simulink model "linear_motor_zs"  (R2017b)
settings: Solver=FixedStepAuto  StartTime=0.0  StopTime=200  FixedStep=1e-3  RelTol=1e-3
values from neighbouring files (symbols this model uses):
  J_ind = 4.1    [linear_motor_params.m]    (also in robust_linear_motor_params.m = ureal('J_ind',4.1,'Percentage',range); ship_induction_motor_propulsion_extended_linear.m)
  L_ad_ind = L_aq_ind    (= 0.00307086614173)    [linear_motor_params.m]    (also in robust_linear_motor_params.m = L_aq_ind; ship_induction_motor_propulsion_extended_linear.m)
  L_aq_ind = 1/(1/L_M_ind + 1/L_ls_ind + 1/L_lr_ind)    (= 0.00307086614173)    [linear_motor_params.m]    (also in robust_linear_motor_params.m = 1/(1/L_M_ind + 1/L_ls_ind + 1/L_lr_ind); ship_induction_motor_propulsion_extended_linear.m)
  L_eq = L_ls_ind + L_M_ind *(L_lr_ind)/(L_lr_ind+L_M_ind)    (= 0.0188613861386)    [linear_motor_params.m]    (also in robust_linear_motor_params.m = L_ls_ind + L_M_ind *(L_lr_ind)/(L_lr_ind+L_M_ind); ship_induction_motor_propulsion_extended_linear.m)
  L_lr_ind = 15e-3    (= 0.015)    [linear_motor_params.m]    (also in robust_linear_motor_params.m = ureal('L_lr_ind',15e-3, 'Percentage',range); ship_induction_motor_propulsion_extended_linear.m)
  L_ls_ind = 15e-3    (= 0.015)    [linear_motor_params.m]    (also in robust_linear_motor_params.m = ureal('L_ls_ind',15e-3, 'Percentage',range); ship_induction_motor_propulsion_extended_linear.m)
  L_M_ind = 5.2e-3    (= 0.0052)    [linear_motor_params.m]    (also in robust_linear_motor_params.m = ureal('L_M_ind',5.2e-3, 'Percentage',range); ship_induction_motor_propulsion_extended_linear.m)
  P_ind = 4    [linear_motor_params.m]    (also in robust_linear_motor_params.m; ship_induction_motor_propulsion_extended_linear.m)
  r_r_ind = 4.6e-3    (= 0.0046)    [linear_motor_params.m]    (also in robust_linear_motor_params.m = ureal('r_r_ind', 4.6e-3, 'Percentage', range); ship_induction_motor_propulsion_extended_linear.m)
  r_s_ind = 7.6e-3    (= 0.0076)    [linear_motor_params.m]    (also in robust_linear_motor_params.m = ureal('r_s_ind', 7.6e-3, 'Percentage', range); ship_induction_motor_propulsion_extended_linear.m)
  T_r_ind = L_lr_ind/r_r_ind    (= 3.26086956522)    [linear_motor_params.m]    (also in robust_linear_motor_params.m = L_lr_ind/r_r_ind; ship_induction_motor_propulsion_extended_linear.m)
  T_s_est = 1e-2    (= 0.01)    [linear_motor_params.m]    (also in robust_linear_motor_params.m; ship_induction_motor_propulsion_extended_linear.m)
  Ts = 1e-3    (= 0.001)    [linear_motor_params.m]    (also in robust_linear_motor_params.m; ship_induction_motor_propulsion_extended_linear.m)
libraries: simulink x6, cstblocks x2
settings Model: Creator=z003vh9b  LastModifiedBy=zhensong
settings CodeAppCC: StateflowObjectComments=on

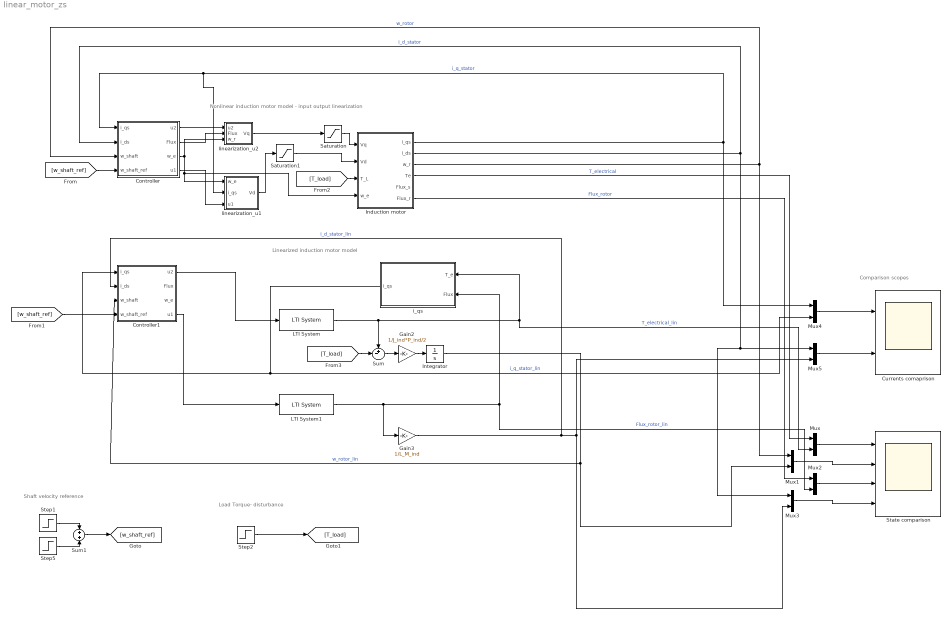
== system linear_motor_zs ==
  note: Comparison scopes
  note: Linearized induction motor model
  note: Nonlinear induction motor model - input output linearization
  note: Load Torque- disturbance
  note: Shaft velocity reference
  Controller : Subsystem
  Controller1 : Subsystem
  Currents comaprison : Scope  NumInputPorts=2
  Gain2 : Gain  Gain=1/J_ind*P_ind/2
  Gain3 : Gain  Gain=1/L_M_ind
  Induction motor : Subsystem
  Integrator : Integrator
  LTI System : cstblocks/LTI System  sys=G_torque  IC=[]  mask(LTI Block){}
  LTI System1 : cstblocks/LTI System  sys=G_flux  IC=[]
  Mux{,1..5} (6 alike) : Mux  Inputs=2
  Saturation : Saturate  UpperLimit=500  LowerLimit=-500
  Saturation1 : Saturate  UpperLimit=500  LowerLimit=-500
  State comparison : Scope  NumInputPorts=4
  Step1 : Step  Time=50  SampleTime=0
  Step2 : Step  Time=100  After=10  SampleTime=0
  Step5 : Step  Time=180  After=-2  SampleTime=0
  Sum : Sum  Inputs=+-|
  Sum1 : Sum
  i_qs : Subsystem
  linearization_u1 : Subsystem
  linearization_u2 : Subsystem
  wires:
  Induction motor/3(w_r) -> Mux1/1, Controller/3(w_shaft)  "w_rotor"
  Induction motor/4(Te) -> Mux/1  "T_electrical"
  Induction motor/2(i_ds) -> Mux3/1, Mux5/1, Controller/2(i_ds)  "i_d_stator"
  Induction motor/1(i_qs) -> Mux4/1, linearization_u1/2(i_qs), Controller/1(i_qs)  "i_q_stator"
  linearization_u2/1(Vq) -> Saturation/1
  linearization_u1/1(Vd) -> Saturation1/1
  Mux/1 -> State comparison/1
  Mux1/1 -> State comparison/2
  Mux2/1 -> State comparison/3
  Mux3/1 -> State comparison/4
  LTI System1/1 -> i_qs/2(Flux), Mux2/2, Gain3/1  "Flux_rotor_lin"
  Gain3/1 -> Mux3/2, Mux5/2, Controller1/2(i_ds)  "i_d_stator_lin"
  Induction motor/6(Flux_r) -> Mux2/1  "Flux_rotor"
  Step5/1 -> Sum1/2
  Step1/1 -> Sum1/1
  [w_shaft_ref] -> Controller/4(w_shaft_ref)
  Saturation/1 -> Induction motor/1(Vq)
  Saturation1/1 -> Induction motor/2(Vd)
  LTI System/1 -> Sum/1, i_qs/1(T_e), Mux/2  "T_electrical_lin"
  Integrator/1 -> Mux1/2, Controller1/3(w_shaft)  "w_rotor_lin"
  Gain2/1 -> Integrator/1
  Controller/1(u2) -> linearization_u2/1(u2)
  Controller/2(Flux) -> linearization_u2/2(Flux)
  Controller/3(w_e) -> linearization_u2/3(w_r), linearization_u1/1(w_e), Induction motor/4(w_e)
  Controller/4(u1) -> linearization_u1/3(u1)
  Controller1/4(u1) -> LTI System1/1
  Controller1/1(u2) -> LTI System/1
  i_qs/1(i_qs) -> Controller1/1(i_qs), Mux4/2  "i_q_stator_lin"
  Sum1/1 -> [w_shaft_ref]
  [w_shaft_ref] -> Controller1/4(w_shaft_ref)
  Step2/1 -> [T_load]
  [T_load] -> Induction motor/3(T_L)
  [T_load] -> Sum/2
  Sum/1 -> Gain2/1
  Mux4/1 -> Currents comaprison/1
  Mux5/1 -> Currents comaprison/2

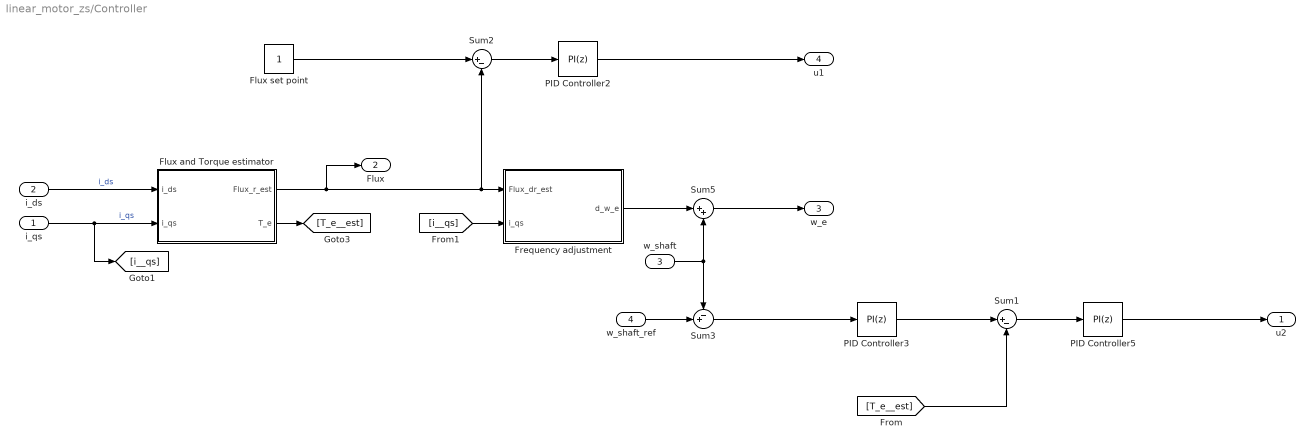
== system linear_motor_zs/Controller ==
  i_qs : Inport
  i_ds : Inport  Port=2
  w_shaft : Inport  Port=3
  w_shaft_ref : Inport  Port=4
  Flux and Torque estimator : Subsystem
  Flux set point : Constant
  Frequency adjustment : Subsystem
  PID Controller2 : simulink/Continuous/PID Controller  Controller=PI  TimeDomain=Discrete-time  SampleTime=0.01  IntegratorMethod=Forward Euler  FilterMethod=Forward Euler  Form=Parallel  UseFilter=on  ControllerParametersSource=internal  P=1  I=0.1  D=0  N=100  InitialConditionSource=internal  InitialConditionForIntegrator=0  InitialConditionForFilter=0  ExternalReset=none  LimitOutput=off  UpperSaturationLimit=inf  LowerSaturationLimit=-inf  LinearizeAsGain=on  AntiWindupMode=none  Kb=1  TrackingMode=off  Kt=1  PParamMin=[]  PParamMax=[]  IParamMin=[]  IParamMax=[]  DParamMin=[]  DParamMax=[]  NParamMin=[]  NParamMax=[]  KbParamMin=[]  KbParamMax=[]  KtParamMin=[]  KtParamMax=[]  POutMin=[]  POutMax=[]  IOutMin=[]  IOutMax=[]  DOutMin=[]  DOutMax=[]  NOutMin=[]  NOutMax=[]  KbOutMin=[]  KbOutMax=[]  KtOutMin=[]  KtOutMax=[]  IntegratorOutMin=[]  IntegratorOutMax=[]  FilterOutMin=[]  FilterOutMax=[]  SumOutMin=[]  SumOutMax=[]  SumI1OutMin=[]  SumI1OutMax=[]  SumI2OutMin=[]  SumI2OutMax=[]  SumI3OutMin=[]  SumI3OutMax=[]  SumDOutMin=[]  SumDOutMax=[]  SaturationOutMin=[]  SaturationOutMax=[]  IntegratorContinuousStateAttributes=''  IntegratorStateMustResolveToSignalObject=off  IntegratorRTWStateStorageClass=Auto  FilterContinuousStateAttributes=''  FilterStateMustResolveToSignalObject=off  FilterRTWStateStorageClass=Auto  DifferentiatorICPrevScaledInput=0  DifferentiatorOutMin=[]  DifferentiatorOutMax=[]  InitialConditionSetting=State (most efficient)  FilterDiffOutCoefMin=[]  FilterDiffOutCoefMax=[]  SumDenOutMin=[]  SumDenOutMax=[]  SumNumOutMin=[]  SumNumOutMax=[]  ReciprocalOutMin=[]  ReciprocalOutMax=[]  DivideOutMin=[]  DivideOutMax=[]  TunerSelectOption=Transfer Function Based (PID Tuner App)
  PID Controller3 : simulink/Continuous/PID Controller  Controller=PI  TimeDomain=Discrete-time  SampleTime=Ts  IntegratorMethod=Forward Euler  FilterMethod=Forward Euler  Form=Parallel  UseFilter=on  ControllerParametersSource=internal  P=10  I=10  D=1  N=100  InitialConditionSource=internal  InitialConditionForIntegrator=0  InitialConditionForFilter=0  ExternalReset=none  LimitOutput=off  UpperSaturationLimit=inf  LowerSaturationLimit=-inf  LinearizeAsGain=on  AntiWindupMode=none  Kb=1  TrackingMode=off  Kt=1  PParamMin=[]  PParamMax=[]  IParamMin=[]  IParamMax=[]  DParamMin=[]  DParamMax=[]  NParamMin=[]  NParamMax=[]  KbParamMin=[]  KbParamMax=[]  KtParamMin=[]  KtParamMax=[]  POutMin=[]  POutMax=[]  IOutMin=[]  IOutMax=[]  DOutMin=[]  DOutMax=[]  NOutMin=[]  NOutMax=[]  KbOutMin=[]  KbOutMax=[]  KtOutMin=[]  KtOutMax=[]  IntegratorOutMin=[]  IntegratorOutMax=[]  FilterOutMin=[]  FilterOutMax=[]  SumOutMin=[]  SumOutMax=[]  SumI1OutMin=[]  SumI1OutMax=[]  SumI2OutMin=[]  SumI2OutMax=[]  SumI3OutMin=[]  SumI3OutMax=[]  SumDOutMin=[]  SumDOutMax=[]  SaturationOutMin=[]  SaturationOutMax=[]  IntegratorContinuousStateAttributes=''  IntegratorStateMustResolveToSignalObject=off  IntegratorRTWStateStorageClass=Auto  FilterContinuousStateAttributes=''  FilterStateMustResolveToSignalObject=off  FilterRTWStateStorageClass=Auto  DifferentiatorICPrevScaledInput=0  DifferentiatorOutMin=[]  DifferentiatorOutMax=[]  InitialConditionSetting=State (most efficient)  FilterDiffOutCoefMin=[]  FilterDiffOutCoefMax=[]  SumDenOutMin=[]  SumDenOutMax=[]  SumNumOutMin=[]  SumNumOutMax=[]  ReciprocalOutMin=[]  ReciprocalOutMax=[]  DivideOutMin=[]  DivideOutMax=[]  TunerSelectOption=Transfer Function Based (PID Tuner App)
  PID Controller5 : simulink/Continuous/PID Controller  Controller=PI  TimeDomain=Discrete-time  SampleTime=Ts  IntegratorMethod=Forward Euler  FilterMethod=Forward Euler  Form=Parallel  UseFilter=on  ControllerParametersSource=internal  P=1  I=10  D=1  N=100  InitialConditionSource=internal  InitialConditionForIntegrator=0  InitialConditionForFilter=0  ExternalReset=none  LimitOutput=off  UpperSaturationLimit=500  LowerSaturationLimit=-500  LinearizeAsGain=on  AntiWindupMode=none  Kb=1  TrackingMode=off  Kt=1  PParamMin=[]  PParamMax=[]  IParamMin=[]  IParamMax=[]  DParamMin=[]  DParamMax=[]  NParamMin=[]  NParamMax=[]  KbParamMin=[]  KbParamMax=[]  KtParamMin=[]  KtParamMax=[]  POutMin=[]  POutMax=[]  IOutMin=[]  IOutMax=[]  DOutMin=[]  DOutMax=[]  NOutMin=[]  NOutMax=[]  KbOutMin=[]  KbOutMax=[]  KtOutMin=[]  KtOutMax=[]  IntegratorOutMin=[]  IntegratorOutMax=[]  FilterOutMin=[]  FilterOutMax=[]  SumOutMin=[]  SumOutMax=[]  SumI1OutMin=[]  SumI1OutMax=[]  SumI2OutMin=[]  SumI2OutMax=[]  SumI3OutMin=[]  SumI3OutMax=[]  SumDOutMin=[]  SumDOutMax=[]  SaturationOutMin=[]  SaturationOutMax=[]  IntegratorContinuousStateAttributes=''  IntegratorStateMustResolveToSignalObject=off  IntegratorRTWStateStorageClass=Auto  FilterContinuousStateAttributes=''  FilterStateMustResolveToSignalObject=off  FilterRTWStateStorageClass=Auto  DifferentiatorICPrevScaledInput=0  DifferentiatorOutMin=[]  DifferentiatorOutMax=[]  InitialConditionSetting=State (most efficient)  FilterDiffOutCoefMin=[]  FilterDiffOutCoefMax=[]  SumDenOutMin=[]  SumDenOutMax=[]  SumNumOutMin=[]  SumNumOutMax=[]  ReciprocalOutMin=[]  ReciprocalOutMax=[]  DivideOutMin=[]  DivideOutMax=[]  TunerSelectOption=Transfer Function Based (PID Tuner App)
  Sum1 : Sum  Inputs=|+-
  Sum2 : Sum  Inputs=|+-
  Sum3 : Sum  Inputs=-+|
  Sum5 : Sum  Inputs=|++
  u2 : Outport
  Flux : Outport  Port=2
  w_e : Outport  Port=3
  u1 : Outport  Port=4
  wires:
  Sum2/1 -> PID Controller2/1
  Sum5/1 -> w_e/1
  Flux and Torque estimator/1(Flux_r_est) -> Flux/1, Frequency adjustment/1(Flux_dr_est), Sum2/2
  w_shaft/1 -> Sum3/1, Sum5/2
  Frequency adjustment/1(d_w_e) -> Sum5/1
  Flux set point/1 -> Sum2/1
  Sum3/1 -> PID Controller3/1
  [i__qs] -> Frequency adjustment/2(i_qs)
  i_ds/1 -> Flux and Torque estimator/1(i_ds)  "i_ds"
  i_qs/1 -> Flux and Torque estimator/2(i_qs), [i__qs]  "i_qs"
  Sum1/1 -> PID Controller5/1
  Flux and Torque estimator/2(T_e) -> [T_e__est]
  PID Controller3/1 -> Sum1/1
  [T_e__est] -> Sum1/2
  PID Controller2/1 -> u1/1
  PID Controller5/1 -> u2/1
  w_shaft_ref/1 -> Sum3/2

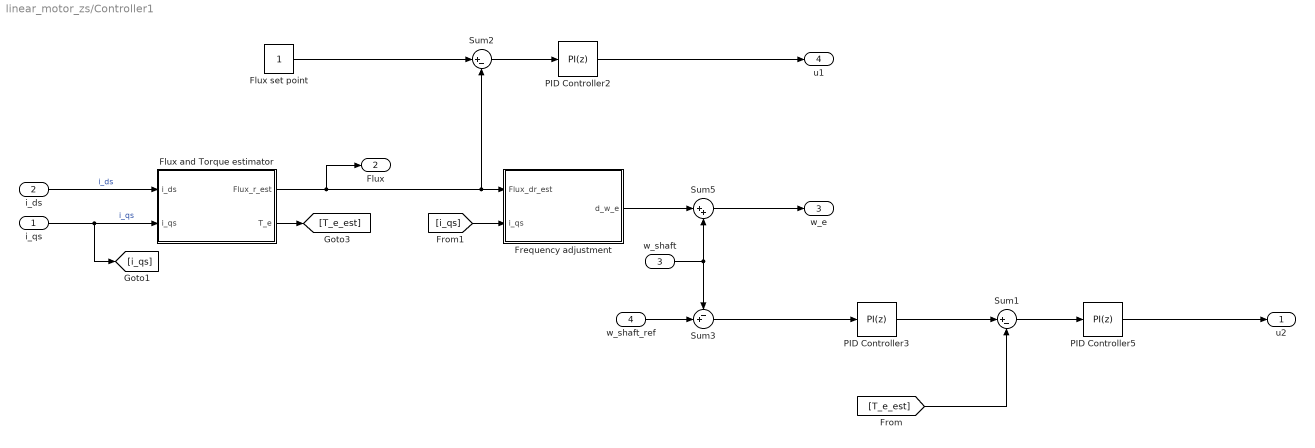
== system linear_motor_zs/Controller1 ==
  i_qs : Inport
  i_ds : Inport  Port=2
  w_shaft : Inport  Port=3
  w_shaft_ref : Inport  Port=4
  Flux and Torque estimator : Subsystem
  Flux set point : Constant
  Frequency adjustment : Subsystem
  PID Controller2 : simulink/Continuous/PID Controller  Controller=PI  TimeDomain=Discrete-time  SampleTime=0.01  IntegratorMethod=Forward Euler  FilterMethod=Forward Euler  Form=Parallel  UseFilter=on  ControllerParametersSource=internal  P=1  I=0.1  D=0  N=100  InitialConditionSource=internal  InitialConditionForIntegrator=0  InitialConditionForFilter=0  ExternalReset=none  LimitOutput=off  UpperSaturationLimit=inf  LowerSaturationLimit=-inf  LinearizeAsGain=on  AntiWindupMode=none  Kb=1  TrackingMode=off  Kt=1  PParamMin=[]  PParamMax=[]  IParamMin=[]  IParamMax=[]  DParamMin=[]  DParamMax=[]  NParamMin=[]  NParamMax=[]  KbParamMin=[]  KbParamMax=[]  KtParamMin=[]  KtParamMax=[]  POutMin=[]  POutMax=[]  IOutMin=[]  IOutMax=[]  DOutMin=[]  DOutMax=[]  NOutMin=[]  NOutMax=[]  KbOutMin=[]  KbOutMax=[]  KtOutMin=[]  KtOutMax=[]  IntegratorOutMin=[]  IntegratorOutMax=[]  FilterOutMin=[]  FilterOutMax=[]  SumOutMin=[]  SumOutMax=[]  SumI1OutMin=[]  SumI1OutMax=[]  SumI2OutMin=[]  SumI2OutMax=[]  SumI3OutMin=[]  SumI3OutMax=[]  SumDOutMin=[]  SumDOutMax=[]  SaturationOutMin=[]  SaturationOutMax=[]  IntegratorContinuousStateAttributes=''  IntegratorStateMustResolveToSignalObject=off  IntegratorRTWStateStorageClass=Auto  FilterContinuousStateAttributes=''  FilterStateMustResolveToSignalObject=off  FilterRTWStateStorageClass=Auto  DifferentiatorICPrevScaledInput=0  DifferentiatorOutMin=[]  DifferentiatorOutMax=[]  InitialConditionSetting=State (most efficient)  FilterDiffOutCoefMin=[]  FilterDiffOutCoefMax=[]  SumDenOutMin=[]  SumDenOutMax=[]  SumNumOutMin=[]  SumNumOutMax=[]  ReciprocalOutMin=[]  ReciprocalOutMax=[]  DivideOutMin=[]  DivideOutMax=[]  TunerSelectOption=Transfer Function Based (PID Tuner App)
  PID Controller3 : simulink/Continuous/PID Controller  Controller=PI  TimeDomain=Discrete-time  SampleTime=Ts  IntegratorMethod=Forward Euler  FilterMethod=Forward Euler  Form=Parallel  UseFilter=on  ControllerParametersSource=internal  P=10  I=10  D=1  N=100  InitialConditionSource=internal  InitialConditionForIntegrator=0  InitialConditionForFilter=0  ExternalReset=none  LimitOutput=off  UpperSaturationLimit=inf  LowerSaturationLimit=-inf  LinearizeAsGain=on  AntiWindupMode=none  Kb=1  TrackingMode=off  Kt=1  PParamMin=[]  PParamMax=[]  IParamMin=[]  IParamMax=[]  DParamMin=[]  DParamMax=[]  NParamMin=[]  NParamMax=[]  KbParamMin=[]  KbParamMax=[]  KtParamMin=[]  KtParamMax=[]  POutMin=[]  POutMax=[]  IOutMin=[]  IOutMax=[]  DOutMin=[]  DOutMax=[]  NOutMin=[]  NOutMax=[]  KbOutMin=[]  KbOutMax=[]  KtOutMin=[]  KtOutMax=[]  IntegratorOutMin=[]  IntegratorOutMax=[]  FilterOutMin=[]  FilterOutMax=[]  SumOutMin=[]  SumOutMax=[]  SumI1OutMin=[]  SumI1OutMax=[]  SumI2OutMin=[]  SumI2OutMax=[]  SumI3OutMin=[]  SumI3OutMax=[]  SumDOutMin=[]  SumDOutMax=[]  SaturationOutMin=[]  SaturationOutMax=[]  IntegratorContinuousStateAttributes=''  IntegratorStateMustResolveToSignalObject=off  IntegratorRTWStateStorageClass=Auto  FilterContinuousStateAttributes=''  FilterStateMustResolveToSignalObject=off  FilterRTWStateStorageClass=Auto  DifferentiatorICPrevScaledInput=0  DifferentiatorOutMin=[]  DifferentiatorOutMax=[]  InitialConditionSetting=State (most efficient)  FilterDiffOutCoefMin=[]  FilterDiffOutCoefMax=[]  SumDenOutMin=[]  SumDenOutMax=[]  SumNumOutMin=[]  SumNumOutMax=[]  ReciprocalOutMin=[]  ReciprocalOutMax=[]  DivideOutMin=[]  DivideOutMax=[]  TunerSelectOption=Transfer Function Based (PID Tuner App)
  PID Controller5 : simulink/Continuous/PID Controller  Controller=PI  TimeDomain=Discrete-time  SampleTime=Ts  IntegratorMethod=Forward Euler  FilterMethod=Forward Euler  Form=Parallel  UseFilter=on  ControllerParametersSource=internal  P=1  I=10  D=1  N=100  InitialConditionSource=internal  InitialConditionForIntegrator=0  InitialConditionForFilter=0  ExternalReset=none  LimitOutput=off  UpperSaturationLimit=500  LowerSaturationLimit=-500  LinearizeAsGain=on  AntiWindupMode=none  Kb=1  TrackingMode=off  Kt=1  PParamMin=[]  PParamMax=[]  IParamMin=[]  IParamMax=[]  DParamMin=[]  DParamMax=[]  NParamMin=[]  NParamMax=[]  KbParamMin=[]  KbParamMax=[]  KtParamMin=[]  KtParamMax=[]  POutMin=[]  POutMax=[]  IOutMin=[]  IOutMax=[]  DOutMin=[]  DOutMax=[]  NOutMin=[]  NOutMax=[]  KbOutMin=[]  KbOutMax=[]  KtOutMin=[]  KtOutMax=[]  IntegratorOutMin=[]  IntegratorOutMax=[]  FilterOutMin=[]  FilterOutMax=[]  SumOutMin=[]  SumOutMax=[]  SumI1OutMin=[]  SumI1OutMax=[]  SumI2OutMin=[]  SumI2OutMax=[]  SumI3OutMin=[]  SumI3OutMax=[]  SumDOutMin=[]  SumDOutMax=[]  SaturationOutMin=[]  SaturationOutMax=[]  IntegratorContinuousStateAttributes=''  IntegratorStateMustResolveToSignalObject=off  IntegratorRTWStateStorageClass=Auto  FilterContinuousStateAttributes=''  FilterStateMustResolveToSignalObject=off  FilterRTWStateStorageClass=Auto  DifferentiatorICPrevScaledInput=0  DifferentiatorOutMin=[]  DifferentiatorOutMax=[]  InitialConditionSetting=State (most efficient)  FilterDiffOutCoefMin=[]  FilterDiffOutCoefMax=[]  SumDenOutMin=[]  SumDenOutMax=[]  SumNumOutMin=[]  SumNumOutMax=[]  ReciprocalOutMin=[]  ReciprocalOutMax=[]  DivideOutMin=[]  DivideOutMax=[]  TunerSelectOption=Transfer Function Based (PID Tuner App)
  Sum1 : Sum  Inputs=|+-
  Sum2 : Sum  Inputs=|+-
  Sum3 : Sum  Inputs=-+|
  Sum5 : Sum  Inputs=|++
  u2 : Outport
  Flux : Outport  Port=2
  w_e : Outport  Port=3
  u1 : Outport  Port=4
  wires:
  Sum2/1 -> PID Controller2/1
  Sum5/1 -> w_e/1
  Flux and Torque estimator/1(Flux_r_est) -> Flux/1, Frequency adjustment/1(Flux_dr_est), Sum2/2
  w_shaft/1 -> Sum3/1, Sum5/2
  Frequency adjustment/1(d_w_e) -> Sum5/1
  Flux set point/1 -> Sum2/1
  Sum3/1 -> PID Controller3/1
  [i_qs] -> Frequency adjustment/2(i_qs)
  i_ds/1 -> Flux and Torque estimator/1(i_ds)  "i_ds"
  i_qs/1 -> Flux and Torque estimator/2(i_qs), [i_qs]  "i_qs"
  Sum1/1 -> PID Controller5/1
  Flux and Torque estimator/2(T_e) -> [T_e_est]
  PID Controller3/1 -> Sum1/1
  [T_e_est] -> Sum1/2
  PID Controller2/1 -> u1/1
  PID Controller5/1 -> u2/1
  w_shaft_ref/1 -> Sum3/2

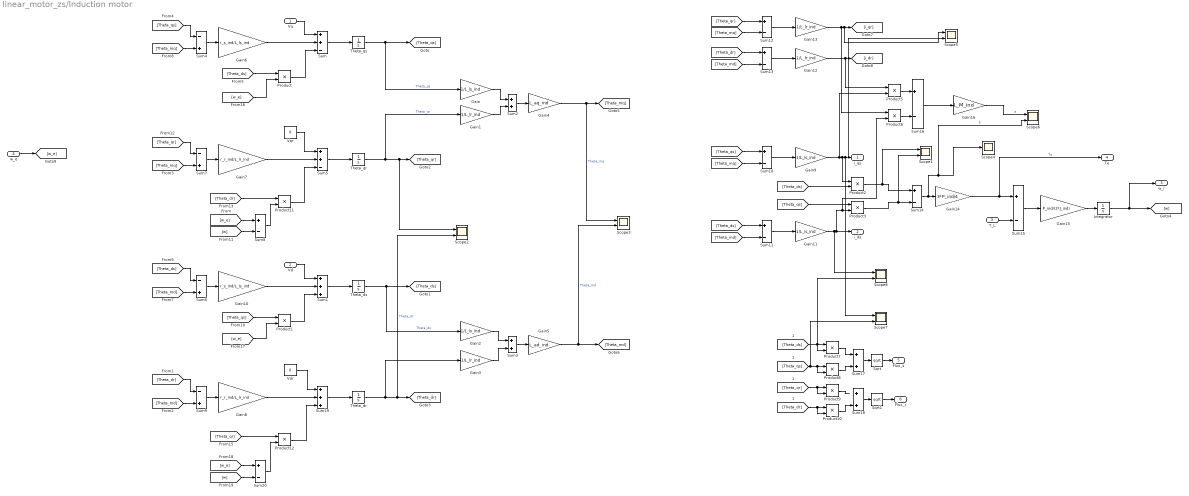
== system linear_motor_zs/Induction motor ==
  Vq : Inport
  Vd : Inport  Port=2
  T_L : Inport  Port=3
  w_e : Inport  Port=4
  Gain{,2,9,11} (4 alike) : Gain  Gain=1/L_ls_ind
  Gain{1,3,12..13} (4 alike) : Gain  Gain=1/L_lr_ind
  Gain10 : Gain  Gain=r_s_ind/L_ls_ind
  Gain14 : Gain  Gain=3*P_ind/4
  Gain15 : Gain  Gain=P_ind/(2*J_ind)
  Gain16 : Gain  Gain=L_M_ind
  Gain4 : Gain  Gain=L_aq_ind
  Gain5 : Gain  Gain=L_ad_ind
  Gain6 : Gain  Gain=r_s_ind/L_ls_ind
  Gain7 : Gain  Gain=r_r_ind/L_lr_ind
  Gain8 : Gain  Gain=r_r_ind/L_lr_ind
  Integrator : Integrator
  Product{,1..3,5..12} (12 alike) : Product
  Scope{1..3,5..8} (7 alike) : Scope  NumInputPorts=2
  Scope4 : Scope
  Sqrt : Sqrt  SaturateOnIntegerOverflow=on
  Sqrt1 : Sqrt  SaturateOnIntegerOverflow=on
  Sum : Sum  Inputs=++-
  Sum1 : Sum  Inputs=+++
  Sum{8,10..16,20} (9 alike) : Sum  Inputs=+-
  Sum{2..3,17..18} (4 alike) : Sum
  Sum19 : Sum  Inputs=+++
  Sum{4,6..7,9} (4 alike) : Sum  Inputs=-+
  Sum5 : Sum  Inputs=++-
  Theta_dr : Integrator
  Theta_ds : Integrator
  Theta_qr : Integrator
  Theta_qs : Integrator
  Vdr : Constant  Value=0
  Vqr : Constant  Value=0
  i_qs : Outport
  i_ds : Outport  Port=2
  w_r : Outport  Port=3
  Te : Outport  Port=4
  Flux_s : Outport  Port=5
  Flux_r : Outport  Port=6
  wires:
  Vq/1 -> Sum/1
  Vd/1 -> Sum1/1
  Sum1/1 -> Theta_ds/1
  Sum/1 -> Theta_qs/1
  Theta_qs/1 -> [Theta_qs], Gain/1  "Theta_qs"
  Theta_ds/1 -> [Theta_ds], Gain2/1  "Theta_ds"
  Theta_qr/1 -> Gain1/1, Scope2/1, [Theta_qr]  "Theta_qr"
  Theta_dr/1 -> Scope2/2, [Theta_dr], Gain3/1  "Theta_dr"
  [Theta_qs] -> Sum4/1
  Sum4/1 -> Gain6/1
  Gain6/1 -> Sum/2
  [Theta_ds] -> Product/1
  Product/1 -> Sum/3
  [w_e] -> Product/2
  [Theta_ds] -> Sum6/1
  Sum6/1 -> Gain10/1
  Gain10/1 -> Sum1/2
  [Theta_qs] -> Product1/1
  [w_e] -> Product1/2
  Product1/1 -> Sum1/3
  Gain/1 -> Sum2/1
  Gain1/1 -> Sum2/2
  Sum2/1 -> Gain4/1
  Gain4/1 -> Scope3/1, [Theta_mq]  "Theta_mq"
  Gain2/1 -> Sum3/1
  Gain3/1 -> Sum3/2
  Sum3/1 -> Gain5/1
  Gain5/1 -> Scope3/2, [Theta_md]  "Theta_md"
  [Theta_mq] -> Sum4/2
  [Theta_md] -> Sum6/2
  Vqr/1 -> Sum5/1
  Sum5/1 -> Theta_qr/1
  [Theta_qr] -> Sum7/1
  Sum7/1 -> Gain7/1
  Gain7/1 -> Sum5/2
  [Theta_mq] -> Sum7/2
  Vdr/1 -> Sum19/1
  Sum19/1 -> Theta_dr/1
  [Theta_dr] -> Sum9/1
  Sum9/1 -> Gain8/1
  Gain8/1 -> Sum19/2
  [Theta_md] -> Sum9/2
  Gain9/1 -> Product5/2, Product2/1, Scope7/1, Scope5/2, i_qs/1
  Gain11/1 -> Scope8/1, Product6/2, Product3/2, i_ds/1
  Sum12/1 -> Gain13/1
  Sum13/1 -> Gain12/1
  [Theta_qs] -> Sum10/1
  [Theta_mq] -> Sum10/2
  [Theta_qr] -> Sum12/1
  [Theta_mq] -> Sum12/2
  [Theta_dr] -> Sum13/1
  [Theta_md] -> Sum13/2
  [Theta_qs] -> Product3/1
  [Theta_ds] -> Product2/2
  Product2/1 -> Scope1/1, Sum14/1
  Product3/1 -> Scope1/2, Sum14/2
  Sum14/1 -> Scope6/2, Scope4/1, Gain14/1  "b"
  Gain14/1 -> Te/1, Sum15/1  "Te"
  T_L/1 -> Sum15/2
  Sum15/1 -> Gain15/1
  Gain15/1 -> Integrator/1
  Integrator/1 -> w_r/1, [w]
  Sum10/1 -> Gain9/1
  [Theta_ds] -> Sum11/1
  [Theta_md] -> Sum11/2
  Sum11/1 -> Gain11/1
  Gain13/1 -> Product6/1, Scope5/1, [i_qr]
  Gain12/1 -> Product5/1, [i_dr]
  Product6/1 -> Sum16/2
  Product5/1 -> Sum16/1
  Gain16/1 -> Scope6/1  "a"
  Sum16/1 -> Gain16/1
  Sqrt/1 -> Flux_s/1
  Sqrt1/1 -> Flux_r/1
  Sum17/1 -> Sqrt/1
  Sum18/1 -> Sqrt1/1
  Product9/1 -> ?
  Product10/1 -> Sum18/2
  Product8/1 -> Sum17/2
  Product7/1 -> Sum17/1
  [Theta_dr] -> Product10/2, Product10/1
  [Theta_qr] -> Product9/1, Product9/2
  [Theta_qs] -> Scope7/2, Product8/2, Product8/1
  [Theta_ds] -> Scope8/2, Product7/2, Product7/1
  [Theta_dr] -> Product11/1
  Product11/1 -> Sum5/3
  [w_e] -> Sum8/1
  [Theta_qr] -> Product12/1
  Product12/1 -> Sum19/3
  w_e/1 -> [w_e]
  [w] -> Sum8/2
  Sum8/1 -> Product11/2
  [w_e] -> Sum20/1
  [w] -> Sum20/2
  Sum20/1 -> Product12/2

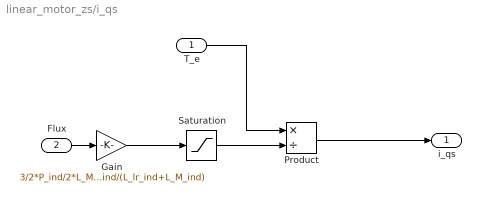
== system linear_motor_zs/i_qs ==
  T_e : Inport
  Flux : Inport  Port=2
  Gain : Gain  Gain=3/2*P_ind/2*L_M_ind/(L_lr_ind+L_M_ind)
  Product : Product  Inputs=*/
  Saturation : Saturate  UpperLimit=inf  LowerLimit=1e-5
  i_qs : Outport
  wires:
  Flux/1 -> Gain/1
  Product/1 -> i_qs/1
  T_e/1 -> Product/1
  Gain/1 -> Saturation/1
  Saturation/1 -> Product/2

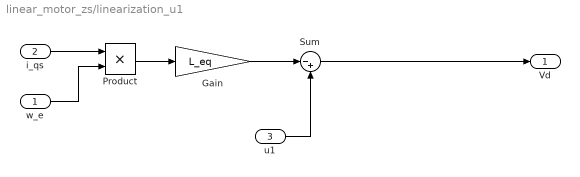
== system linear_motor_zs/linearization_u1 ==
  w_e : Inport
  i_qs : Inport  Port=2
  u1 : Inport  Port=3
  Gain : Gain  Gain=L_eq
  Product : Product
  Sum : Sum  Inputs=|-+
  Vd : Outport
  wires:
  u1/1 -> Sum/2
  i_qs/1 -> Product/1
  w_e/1 -> Product/2
  Product/1 -> Gain/1
  Sum/1 -> Vd/1
  Gain/1 -> Sum/1

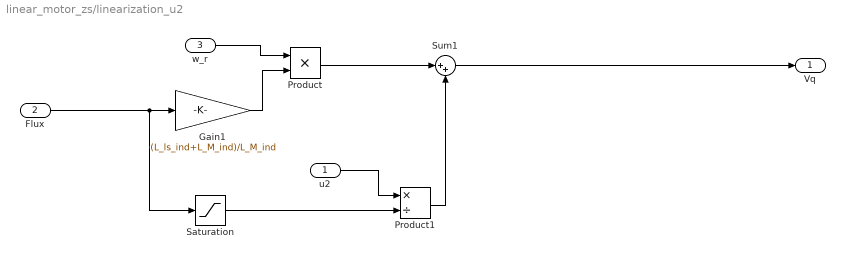
== system linear_motor_zs/linearization_u2 ==
  u2 : Inport
  Flux : Inport  Port=2
  w_r : Inport  Port=3
  Gain1 : Gain  Gain=(L_ls_ind+L_M_ind)/L_M_ind
  Product : Product
  Product1 : Product  Inputs=*/
  Saturation : Saturate  UpperLimit=inf  LowerLimit=1e-5
  Sum1 : Sum  Inputs=|++
  Vq : Outport
  wires:
  Gain1/1 -> Product/2
  Flux/1 -> Saturation/1, Gain1/1
  u2/1 -> Product1/1
  Sum1/1 -> Vq/1
  Product/1 -> Sum1/1
  Product1/1 -> Sum1/2
  Saturation/1 -> Product1/2
  w_r/1 -> Product/1

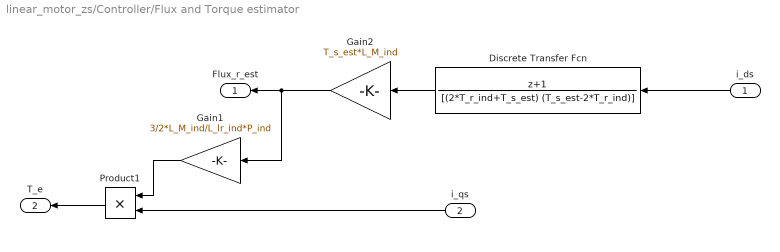
== system linear_motor_zs/Controller/Flux and Torque estimator ==
  i_ds : Inport
  i_qs : Inport  Port=2
  Discrete Transfer Fcn : DiscreteTransferFcn  Numerator=[1 1]  Denominator=[(2*T_r_ind+T_s_est) (T_s_est-2*T_r_ind)]  SampleTime=T_s_est
  Gain1 : Gain  Gain=3/2*L_M_ind/L_lr_ind*P_ind
  Gain2 : Gain  Gain=T_s_est*L_M_ind
  Product1 : Product
  Flux_r_est : Outport
  T_e : Outport  Port=2
  wires:
  i_qs/1 -> Product1/2
  Gain2/1 -> Flux_r_est/1, Gain1/1
  Gain1/1 -> Product1/1
  i_ds/1 -> Discrete Transfer Fcn/1
  Product1/1 -> T_e/1
  Discrete Transfer Fcn/1 -> Gain2/1

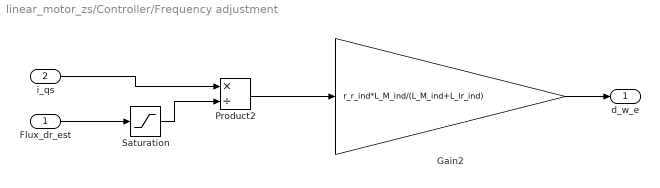
== system linear_motor_zs/Controller/Frequency adjustment ==
  Flux_dr_est : Inport
  i_qs : Inport  Port=2
  Gain2 : Gain  Gain=r_r_ind*L_M_ind/(L_M_ind+L_lr_ind)
  Product2 : Product  Inputs=*/
  Saturation : Saturate  UpperLimit=inf  LowerLimit=1e-5
  d_w_e : Outport
  wires:
  i_qs/1 -> Product2/1
  Product2/1 -> Gain2/1
  Saturation/1 -> Product2/2
  Gain2/1 -> d_w_e/1
  Flux_dr_est/1 -> Saturation/1

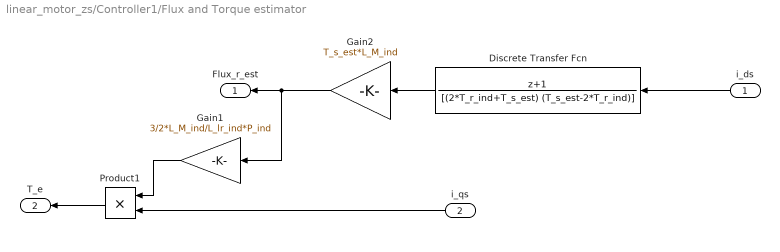
== system linear_motor_zs/Controller1/Flux and Torque estimator ==
  i_ds : Inport
  i_qs : Inport  Port=2
  Discrete Transfer Fcn : DiscreteTransferFcn  Numerator=[1 1]  Denominator=[(2*T_r_ind+T_s_est) (T_s_est-2*T_r_ind)]  SampleTime=T_s_est
  Gain1 : Gain  Gain=3/2*L_M_ind/L_lr_ind*P_ind
  Gain2 : Gain  Gain=T_s_est*L_M_ind
  Product1 : Product
  Flux_r_est : Outport
  T_e : Outport  Port=2
  wires:
  i_qs/1 -> Product1/2
  Gain2/1 -> Flux_r_est/1, Gain1/1
  Gain1/1 -> Product1/1
  i_ds/1 -> Discrete Transfer Fcn/1
  Product1/1 -> T_e/1
  Discrete Transfer Fcn/1 -> Gain2/1

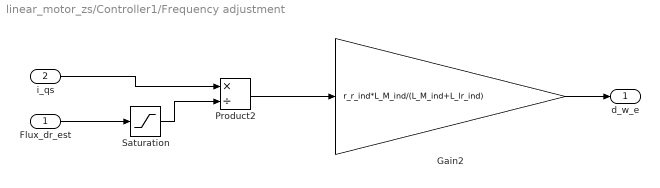
== system linear_motor_zs/Controller1/Frequency adjustment ==
  Flux_dr_est : Inport
  i_qs : Inport  Port=2
  Gain2 : Gain  Gain=r_r_ind*L_M_ind/(L_M_ind+L_lr_ind)
  Product2 : Product  Inputs=*/
  Saturation : Saturate  UpperLimit=inf  LowerLimit=1e-5
  d_w_e : Outport
  wires:
  i_qs/1 -> Product2/1
  Product2/1 -> Gain2/1
  Saturation/1 -> Product2/2
  Gain2/1 -> d_w_e/1
  Flux_dr_est/1 -> Saturation/1
